simulink model "Exo_IMU"  (R2016a)
settings: Solver=FixedStepDiscrete  StartTime=0.0  StopTime=inf  FixedStep=0.2  RelTol=1e-3
undefined symbols (not defined in the file or in its folder): deg, s
libraries: ExoSense_library x5, IMUboard_library x1, QB_pacer_lib x1, qbmove_library x1
settings Model: Creator=laurentio  LastModifiedBy=MattiaCP
settings DataIOCC: LimitDataPoints=on  SaveFormat=Array
settings DebuggingCC: UnderspecifiedInitializationDetection=Classic  MergeDetectMultiDrivingBlocksExec=none  SolverPrmCheckMsg=warning  AllowSymbolicDim=off  StateNameClashWarn=warning
settings HardwareCC: ProdBitPerPointer=32  ProdLargestAtomicFloat=None  ProdIntDivRoundTo=Undefined  ProdEndianess=Unspecified  ProdWordSize=32  ProdHWDeviceType=32-bit Generic
settings ModelReferenceCC: PropagateSignalLabelsOutOfModel=off
settings ConfigComp: CovModelRefEnable=Off  CovSFcnEnable=off

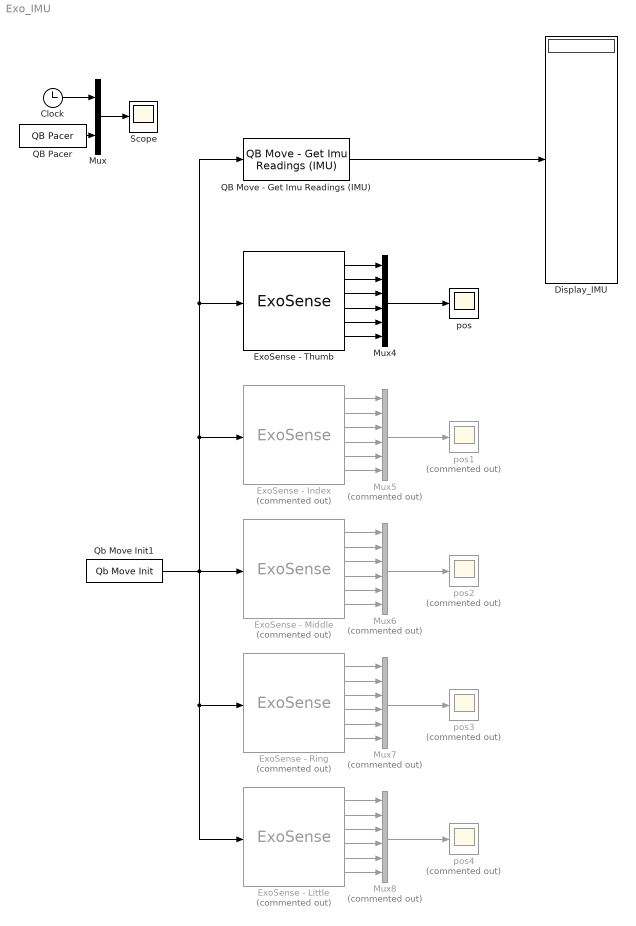
== system Exo_IMU ==
  Clock : Clock
  "Display_IMU " : Display
  ExoSense - Index : ExoSense_library/ExoSense  Commented=on  ID=2  ACTIVE_COMM_DIRECTIONS=Rx  CONTROL_MODE=Prime Movers Positions  DAISY_CHAINING=off  MAX_ANG=0  SW_LIMIT=inf  OFFSET=0  ACTIVATE=off  WDT=0.0  UNITY=Degrees
  ExoSense - Little : ExoSense_library/ExoSense  Commented=on  ID=5  ACTIVE_COMM_DIRECTIONS=Rx  CONTROL_MODE=Prime Movers Positions  DAISY_CHAINING=off  MAX_ANG=0  SW_LIMIT=inf  OFFSET=0  ACTIVATE=off  WDT=0.0  UNITY=Degrees
  ExoSense - Middle : ExoSense_library/ExoSense  Commented=on  ID=3  ACTIVE_COMM_DIRECTIONS=Rx  CONTROL_MODE=Prime Movers Positions  DAISY_CHAINING=off  MAX_ANG=0  SW_LIMIT=inf  OFFSET=0  ACTIVATE=off  WDT=0.0  UNITY=Degrees
  ExoSense - Ring : ExoSense_library/ExoSense  Commented=on  ID=4  ACTIVE_COMM_DIRECTIONS=Rx  CONTROL_MODE=Prime Movers Positions  DAISY_CHAINING=off  MAX_ANG=0  SW_LIMIT=inf  OFFSET=0  ACTIVATE=off  WDT=0.0  UNITY=Degrees
  ExoSense - Thumb : ExoSense_library/ExoSense  ID=1  ACTIVE_COMM_DIRECTIONS=Rx  CONTROL_MODE=Prime Movers Positions  DAISY_CHAINING=off  MAX_ANG=0  SW_LIMIT=inf  OFFSET=0  ACTIVATE=off  WDT=0.0  UNITY=Degrees
  Mux : Mux  Inputs=2
  Mux4 : Mux  Inputs=6
  Mux{5..8} (4 alike) : Mux  Commented=on  Inputs=6
  QB Move - Get Imu Readings (IMU) : IMUboard_library/QB Move - Get Imu Readings (IMU)  ID=6  N_IMU=1  DAISY_CHAINING=off  ACC_UNITY=G  GYRO_UNITY=deg/s  MAG_UNITY=uT
  QB Pacer : QB_pacer_lib/QB Pacer  simTimePerRealTime=1
  Qb Move Init1 : qbmove_library/Qb Move Init  NUMBER_OF_COM='COM5'  BAUD_RATE_COM=2000000
  Scope : Scope
  pos : Scope
  pos{1..4} (4 alike) : Scope  Commented=on
  wires:
  Qb Move Init1/1 -> ExoSense - Middle/1, ExoSense - Little/1, ExoSense - Ring/1, ExoSense - Index/1, QB Move - Get Imu Readings (IMU)/1, ExoSense - Thumb/1
  QB Pacer/1 -> Mux/2
  Clock/1 -> Mux/1
  Mux/1 -> Scope/1
  Mux4/1 -> pos/1
  ExoSense - Thumb/4 -> Mux4/4
  ExoSense - Thumb/3 -> Mux4/3
  ExoSense - Thumb/6 -> Mux4/6
  ExoSense - Thumb/5 -> Mux4/5
  Mux5/1 -> pos1/1
  ExoSense - Index/2 -> Mux5/2
  ExoSense - Index/4 -> Mux5/4
  ExoSense - Index/3 -> Mux5/3
  ExoSense - Index/6 -> Mux5/6
  ExoSense - Index/1 -> Mux5/1
  ExoSense - Index/5 -> Mux5/5
  Mux6/1 -> pos2/1
  ExoSense - Middle/2 -> Mux6/2
  ExoSense - Middle/4 -> Mux6/4
  ExoSense - Middle/3 -> Mux6/3
  ExoSense - Middle/6 -> Mux6/6
  ExoSense - Middle/5 -> Mux6/5
  Mux7/1 -> pos3/1
  ExoSense - Ring/2 -> Mux7/2
  ExoSense - Ring/4 -> Mux7/4
  ExoSense - Ring/3 -> Mux7/3
  ExoSense - Ring/6 -> Mux7/6
  ExoSense - Ring/5 -> Mux7/5
  Mux8/1 -> pos4/1
  ExoSense - Little/2 -> Mux8/2
  ExoSense - Little/4 -> Mux8/4
  ExoSense - Little/3 -> Mux8/3
  ExoSense - Little/6 -> Mux8/6
  ExoSense - Little/5 -> Mux8/5
  ExoSense - Middle/1 -> Mux6/1
  ExoSense - Ring/1 -> Mux7/1
  ExoSense - Little/1 -> Mux8/1
  ExoSense - Thumb/1 -> Mux4/1
  ExoSense - Thumb/2 -> Mux4/2
  QB Move - Get Imu Readings (IMU)/1 -> "Display_IMU "/1
